simulink model "Slip_Brake_Control"  (R2023b)
settings: Solver=VariableStepAuto  StartTime=0.0  StopTime=10.0  RelTol=1e-3
settings Model: Creator=E8KUAVE  LastModifiedBy=E8KUAVE

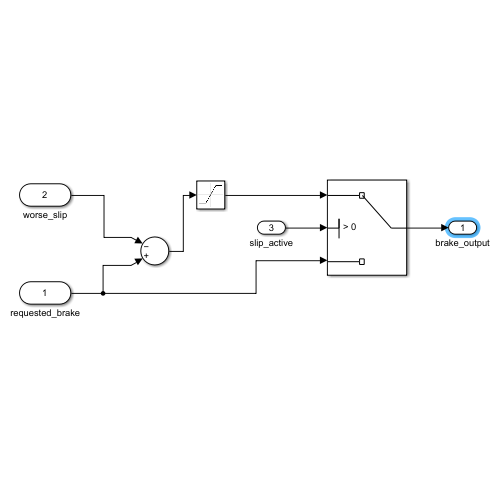
[thumbnail: Simulink's stored preview of the top-level diagram]
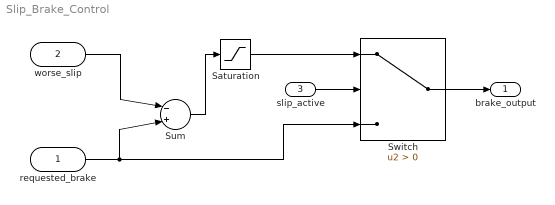
== system Slip_Brake_Control ==
  requested_brake : Inport  OutDataTypeStr=uint16
  worse_slip : Inport  Port=2  OutDataTypeStr=uint16
  slip_active : Inport  Port=3  OutDataTypeStr=boolean
  Saturation : Saturate  UpperLimit=1000  LowerLimit=0  OutDataTypeStr=uint16
  Sum : Sum  Inputs=|-+|  OutDataTypeStr=int16
  Switch : Switch  Criteria=u2 > Threshold  SaturateOnIntegerOverflow=off  InputSameDT=off
  brake_output : Outport  OutDataTypeStr=uint16
  wires:
  worse_slip/1 -> Sum/1
  requested_brake/1 -> Switch/3, Sum/2
  Sum/1 -> Saturation/1
  slip_active/1 -> Switch/2
  Saturation/1 -> Switch/1
  Switch/1 -> brake_output/1
